simulink model "rlOvertakeTwoCars"  (R2022b)
settings: Solver=ode45  StartTime=0.0  StopTime=inf  FixedStep=0.001  RelTol=5e-3
PreLoadFcn:
  | setUpModel
PostLoadFcn:
  | setUpMain
model workspace (MAT data in the model file):
  firstWarning = 0
  originalScenarioChecksum = 'F73A6DA3C723D3CA73A6F931B7A52A9C'
values from neighbouring files (symbols this model uses):
  accel_vec = (-4:0.5:4)'    [setUpModel.m]
  amax = 3    [setUpMain.m]
  amin = -3    [setUpMain.m]
  dyNorm = [dyNorm 1.1]    [setUpSlipstream.m]
  e1_initial = 0    [setUpMain.m]
  e2_initial = 0    [setUpMain.m]
  L = data.ActorSpecifications.Length    [setUpModel.m]
  psi_o1 = 0.0058 * (pi/180)    (= 0.000101229096616)    [setUpModel.m]
  psi_o2 = 0.3528 *(pi/180)    (= 0.00615752160104)    [setUpModel.m]
  ry = [ry 0]    [setUpSlipstream.m]
  ssSwitch = 1    [setUpSlipstream.m]
  tolpsi = 10 * pi/180    (= 0.174532925199)    [setUpSlipstream.m]
  toly = 1.2*W /2    [setUpSlipstream.m]
  Ts = 0.1    [setUpMPC.m]
  TsRL = Ts    [setUpRLEnv.m]
  umax = 0.3    [setUpMain.m]
  umin = -0.3    [setUpMain.m]
  v_o1 = highSpeed1    (= 35)    [setUpModel.m]
  v_o2 = highSpeed2    (= 36)    [setUpModel.m]
  vel1 = highSpeed1 * ones(length(xlt),length(ylt))    [setUpModel.m]
  vel2 = highSpeed2 * ones(length(xlt),length(ylt))    [setUpModel.m]
  vel_vec = 0:2:20    [setUpModel.m]
  W = data.ActorSpecifications(1,1).Width    [setUpSlipstream.m]
  X_o1 = xRef1(1)    [setUpModel.m]
  X_o2 = xRef2(1)    [setUpModel.m]
  xFollow = [0 x1 xFollow 60]    [setUpSlipstream.m]
  xLead = [0 -x0 xLead]    [setUpSlipstream.m]
  xlt = -250:10:200    [setUpModel.m]
  Y_o1 = yRef1(1)    [setUpModel.m]
  Y_o2 = yRef2(1)    [setUpModel.m]
  yFollow = [c y1 yFollow 1]    [setUpSlipstream.m]
  yLead = [c y0 yLead]    [setUpSlipstream.m]
  ylt = -150:10:100    [setUpModel.m]
undefined symbols (not defined in the file or in its folder): curvature1, curvature2, deg, DiscIntNeverNeededParam, gradbp1, gradbp2, psi, rad, s, v_o, x_colpen, x_o, y_colpen, Z_colpen
libraries: simulink x26, autolibsharedcommon x22, autolibutils x10, autolibshared x10, vehdynlibtirecommon x8, drivingscenarioandsensors x4, autolibpowerinfoutils x4, sharedtransform x4, aerolibconvert2 x2, simulink_extras x2, vehdynlibtire x2, mpcadaslib x1
(part 4 of 8)

== system rlOvertakeTwoCars/Vehicle Body 3DOF Dual Track/sigma ==
  note: 1) Add Subsystem or Model blocks as valid variant choices.
      | 2) You cannot connect blocks at this level. At simulation, connectivity is automatically
      | determined, based on the active variant and port name matching.
  y : Inport
  no sigma : Subsystem  VariantControl=0
  no sigma dual : Subsystem  VariantControl=2
  sigma : Subsystem  VariantControl=1
  sigma dual : Subsystem  VariantControl=3
  alpha_f : Outport  VectorParamsAs1DForOutWhenUnconnected=off
  alpha_r : Outport  Port=2  VectorParamsAs1DForOutWhenUnconnected=off

== system rlOvertakeTwoCars/Vehicle Body 3DOF Dual Track/state ==
  note: 1) Add Subsystem or Model blocks as valid variant choices.
      | 2) You cannot connect blocks at this level. At simulation, connectivity is automatically
      | determined, based on the active variant and port name matching.
  xdot : Inport  Unit=m/s
  xddot_in : Inport  Port=2  PortDimensions=4
  extState : Inport  Port=3
  xdot ext : Subsystem  VariantControl=1
  xdot int : Subsystem  VariantControl=0
  xddot_out : Outport  VectorParamsAs1DForOutWhenUnconnected=off

== system rlOvertakeTwoCars/Vehicle Body 3DOF Dual Track/wind ==
  note: 1) Add Subsystem or Model blocks as valid variant choices.
      | 2) You cannot connect blocks at this level. At simulation, connectivity is automatically
      | determined, based on the active variant and port name matching.
  wind_in : Inport  Unit=m/s
  wind ext : Subsystem  VariantControl=1
  wind int : Subsystem  VariantControl=0
  wind_out : Outport  Unit=m/s  VectorParamsAs1DForOutWhenUnconnected=off

== system rlOvertakeTwoCars/Vehicle Body 3DOF Dual Track Ego/Cy ==
  note: 1) Add Subsystem or Model blocks as valid variant choices.
      | 2) You cannot connect blocks at this level. At simulation, connectivity is automatically
      | determined, based on the active variant and port name matching.
  alpha_f : Inport
  alpha_r : Inport  Port=2
  Cy const : Subsystem  VariantControl=0
  Cy const dual : Subsystem  VariantControl=2
  Cy table : Subsystem  VariantControl=1
  Cy table dual : Subsystem  VariantControl=3
  Cy_f : Outport  VectorParamsAs1DForOutWhenUnconnected=off
  Cy_r : Outport  Port=2  VectorParamsAs1DForOutWhenUnconnected=off

== system rlOvertakeTwoCars/Vehicle Body 3DOF Dual Track Ego/Drag ==
  wind : Inport
  y : Inport  Port=2
  Temp : Inport  Port=3  Unit=K
  Constant : Constant  Value=0
  Demux : Demux  Outputs=3
  Drag Force : autolibsharedcommon/Vehicle Body 3dof/Drag Force  A=Af  beta_w=beta_w  Cd=Cd  Cs=Cs  Cl=Cl  Cpm=Cpm  Lcpm=a+b  Crm=beta_w.*0  Cym=Cym  R=287.058  Pabs=Pabs
  Selector2 : Selector  InputPortWidth=4  IndexOptions=Index vector (dialog)  Indices=[1:3]  OutputSizes=1
  Unary Minus : UnaryMinus
  Unary Minus1 : UnaryMinus
  Vector Concatenate1 : Concatenate  NumInputs=3
  inertial2body : Subsystem
  Fd : Outport  VectorParamsAs1DForOutWhenUnconnected=off
  Md : Outport  Port=2  VectorParamsAs1DForOutWhenUnconnected=off
  wires:
  Temp/1 -> Drag Force/3
  inertial2body/1(Windxyz) -> Drag Force/2
  wind/1 -> inertial2body/2(WindXYZ)
  Demux/3 -> inertial2body/1(psi)
  Demux/1 -> Vector Concatenate1/1
  Demux/2 -> Vector Concatenate1/2
  Constant/1 -> Vector Concatenate1/3
  Vector Concatenate1/1 -> Drag Force/1
  Selector2/1 -> Demux/1
  Drag Force/2 -> Unary Minus1/1
  y/1 -> Selector2/1
  Drag Force/1 -> Unary Minus/1
  Unary Minus/1 -> Fd/1
  Unary Minus1/1 -> Md/1

== system rlOvertakeTwoCars/Vehicle Body 3DOF Dual Track Ego/Signal Routing ==
  note: 1) Add Subsystem or Model blocks as valid variant choices.
      | 2) You cannot connect blocks at this level. At simulation, connectivity is automatically
      | determined, based on the active variant and port name matching.
  y : Inport
  Fbody : Inport  Port=2  Unit=N
  MTotal : Inport  Port=3  Unit=N*m
  FOut : Inport  Port=4
  FTire : Inport  Port=5  Unit=N
  Fg : Inport  Port=6  Unit=N
  FDrag : Inport  Port=7  Unit=N
  MDrag : Inport  Port=8  Unit=N*m
  FExt : Inport  Port=9  Unit=N
  MExt : Inport  Port=10  Unit=N*m
  x : Inport  Port=11
  WhlAngF : Inport  Port=12
  WhlAngR : Inport  Port=13
  Fh : Inport  Port=14  Unit=N
  Mh : Inport  Port=15  Unit=N*m
  Xo : Inport  Port=16
  Signal Routing : Subsystem  VariantControl=0
  Signal Routing Dual : Subsystem  VariantControl=1
  Info : Outport  VectorParamsAs1DForOutWhenUnconnected=off
  xdot : Outport  Port=2  VectorParamsAs1DForOutWhenUnconnected=off
  ydot : Outport  Port=3  VectorParamsAs1DForOutWhenUnconnected=off
  psi : Outport  Port=4  VectorParamsAs1DForOutWhenUnconnected=off
  r : Outport  Port=5  VectorParamsAs1DForOutWhenUnconnected=off
  FzF : Outport  Port=6  VectorParamsAs1DForOutWhenUnconnected=off
  FzR : Outport  Port=7  VectorParamsAs1DForOutWhenUnconnected=off

== system rlOvertakeTwoCars/Vehicle Body 3DOF Dual Track Ego/Slipstream drag multiplier ==
  note: Switch
  note: Lateral offset effect
  note: Drag coefficient ratio
  G : Inport
  Add : Sum  Inputs=-++
  Constant : Constant
  Constant1 : Constant
  "G<0, following" : Lookup_n-D  NumberOfTableDimensions=1  BreakpointsForDimension1=xFollow  Table=yFollow  InternalRulePriority=Speed  RndMeth=Simplest
  "G>0, leading" : Lookup_n-D  NumberOfTableDimensions=1  BreakpointsForDimension1=xLead  Table=yLead  InternalRulePriority=Speed  RndMeth=Simplest
  Lateral multiplier : Lookup_n-D  NumberOfTableDimensions=1  BreakpointsForDimension1=dyNorm  Table=ry  InternalRulePriority=Speed  RndMeth=Simplest
  Multiply : Gain  Gain=-1
  Product : Product
  Switch : Switch  Criteria=u2 > Threshold  SaturateOnIntegerOverflow=off  InputSameDT=off
  Switch1 : Switch  Criteria=u2 > Threshold  SaturateOnIntegerOverflow=off  InputSameDT=off
  r_Cd' : Outport
  tag scope: ry2=global
  wires:
  G/1 -> "G>0, leading"/1, Switch/2, Multiply/1
  "G>0, leading"/1 -> Switch/1
  "G<0, following"/1 -> Switch/3
  Multiply/1 -> "G<0, following"/1
  Constant/1 -> Switch1/3
  Switch1/1 -> r_Cd'/1
  [SsOn] -> Switch1/2
  [dyNorm] -> Lateral multiplier/1
  Switch/1 -> Product/2  "r_Cd"
  Lateral multiplier/1 -> [ry2], Add/1, Product/1  "ry"
  Product/1 -> Add/2
  Constant1/1 -> Add/3
  Add/1 -> Switch1/1

== system rlOvertakeTwoCars/Vehicle Body 3DOF Dual Track Ego/friction ==
  note: 1) Add Subsystem or Model blocks as valid variant choices.
      | 2) You cannot connect blocks at this level. At simulation, connectivity is automatically
      | determined, based on the active variant and port name matching.
  mu_in : Inport  Unit=1
  mu ext : Subsystem  VariantControl=1
  mu ext dual : Subsystem  VariantControl=3
  mu int : Subsystem  VariantControl=0
  mu int dual : Subsystem  VariantControl=2
  mu_out : Outport  Unit=1  VectorParamsAs1DForOutWhenUnconnected=off

== system rlOvertakeTwoCars/Vehicle Body 3DOF Dual Track Ego/front forces ==
  note: 1) Add Subsystem or Model blocks as valid variant choices.
      | 2) You cannot connect blocks at this level. At simulation, connectivity is automatically
      | determined, based on the active variant and port name matching.
  F_in : Inport  Unit=N
  ext : Subsystem  VariantControl=2
  ext dual : Subsystem  VariantControl=5
  ext long : Subsystem  VariantControl=1
  ext long dual : Subsystem  VariantControl=4
  int : Subsystem  VariantControl=0
  int dual : Subsystem  VariantControl=3
  F_out : Outport  Unit=N  VectorParamsAs1DForOutWhenUnconnected=off

== system rlOvertakeTwoCars/Vehicle Body 3DOF Dual Track Ego/front steer ==
  note: 1) Add Subsystem or Model blocks as valid variant choices.
      | 2) You cannot connect blocks at this level. At simulation, connectivity is automatically
      | determined, based on the active variant and port name matching.
  delta_in : Inport  Unit=rad
  delta ext : Subsystem  VariantControl=1
  delta ext dual : Subsystem  VariantControl=3
  delta int : Subsystem  VariantControl=0
  delta int dual : Subsystem  VariantControl=2
  delta_out : Outport  Unit=rad  VectorParamsAs1DForOutWhenUnconnected=off

== system rlOvertakeTwoCars/Vehicle Body 3DOF Dual Track Ego/hitch geometry parameters ==
  note: 1) Add Subsystem or Model blocks as valid variant choices.
      | 2) You cannot connect blocks at this level. At simulation, connectivity is automatically
      | determined, based on the active variant and port name matching.
  hitch active bicycle : Subsystem  VariantControl=1
  hitch active dual track : Subsystem  VariantControl=2
  hitch inactive : Subsystem  VariantControl=3
  dh_out : Outport  Unit=m  VectorParamsAs1DForOutWhenUnconnected=off
  hl_out : Outport  Port=2  Unit=m  VectorParamsAs1DForOutWhenUnconnected=off
  hh_out : Outport  Port=3  Unit=m  VectorParamsAs1DForOutWhenUnconnected=off

== system rlOvertakeTwoCars/Vehicle Body 3DOF Dual Track Ego/sigma ==
  note: 1) Add Subsystem or Model blocks as valid variant choices.
      | 2) You cannot connect blocks at this level. At simulation, connectivity is automatically
      | determined, based on the active variant and port name matching.
  y : Inport
  no sigma : Subsystem  VariantControl=0
  no sigma dual : Subsystem  VariantControl=2
  sigma : Subsystem  VariantControl=1
  sigma dual : Subsystem  VariantControl=3
  alpha_f : Outport  VectorParamsAs1DForOutWhenUnconnected=off
  alpha_r : Outport  Port=2  VectorParamsAs1DForOutWhenUnconnected=off

== system rlOvertakeTwoCars/Vehicle Body 3DOF Dual Track Ego/state ==
  note: 1) Add Subsystem or Model blocks as valid variant choices.
      | 2) You cannot connect blocks at this level. At simulation, connectivity is automatically
      | determined, based on the active variant and port name matching.
  xdot : Inport  Unit=m/s
  xddot_in : Inport  Port=2  PortDimensions=4
  extState : Inport  Port=3
  xdot ext : Subsystem  VariantControl=1
  xdot int : Subsystem  VariantControl=0
  xddot_out : Outport  VectorParamsAs1DForOutWhenUnconnected=off

== system rlOvertakeTwoCars/Vehicle Body 3DOF Dual Track Ego/wind ==
  note: 1) Add Subsystem or Model blocks as valid variant choices.
      | 2) You cannot connect blocks at this level. At simulation, connectivity is automatically
      | determined, based on the active variant and port name matching.
  wind_in : Inport  Unit=m/s
  wind ext : Subsystem  VariantControl=1
  wind int : Subsystem  VariantControl=0
  wind_out : Outport  Unit=m/s  VectorParamsAs1DForOutWhenUnconnected=off

== system rlOvertakeTwoCars/Powertrain & Driveline/Brakes and Wheels/Whl2Veh ==
  FxWhlFrm : Inport  PortDimensions=4
  FyWhlFrm : Inport  Port=2  PortDimensions=4
  WhlAng : Inport  Port=3
  Add : Sum  Inputs=+-
  Add1 : Sum
  Demux2 : Demux  Outputs=[2 2]
  Demux3 : Demux  Outputs=[2 2]
  Product{1..4} (4 alike) : Product
  SinCos : Trigonometry  Operator=sincos
  Vector Concatenate : Concatenate  Mode=Multidimensional array  ConcatenateDimension=2
  Vector Concatenate1 : Concatenate  Mode=Multidimensional array  ConcatenateDimension=2
  FrontF : Outport
  RearF : Outport  Port=2
  wires:
  Vector Concatenate/1 -> FrontF/1
  Demux3/1 -> Vector Concatenate/2
  Demux2/1 -> Vector Concatenate/1
  Demux2/2 -> Vector Concatenate1/1
  Demux3/2 -> Vector Concatenate1/2
  Vector Concatenate1/1 -> RearF/1
  Product4/1 -> Add1/2
  Add/1 -> Demux2/1
  Product2/1 -> Add/2
  SinCos/1 -> Product2/2, Product3/2
  Product1/1 -> Add/1
  SinCos/2 -> Product4/2, Product1/2
  FyWhlFrm/1 -> Product4/1, Product2/1
  Add1/1 -> Demux3/1
  FxWhlFrm/1 -> Product3/1, Product1/1
  Product3/1 -> Add1/1
  WhlAng/1 -> SinCos/1

== system rlOvertakeTwoCars/Powertrain & Driveline/Brakes and Wheels/scale factors with friction ==
  lamda_mu_x : Inport
  lamda_mu_y : Inport  Port=2
  0 : Constant  Value=[zeros(1,numWheels)]  VectorParams1D=off
  Reshape : Reshape  OutputDimensionality=Row vector (2-D)  OutputDimensions=[1,numWheels]
  Reshape1 : Reshape  OutputDimensionality=Row vector (2-D)  OutputDimensions=[1,numWheels]
  Signal Specification3 : SignalSpecification  Unit=1
  Vector Concatenate : Concatenate  NumInputs=5  Mode=Multidimensional array
  ones : Constant  Value=[ones(23,numWheels)]  VectorParams1D=off
  ones2 : Constant  Value=ones(1,numWheels)  VectorParams1D=off
  lambdas : Outport  Unit=1  VectorParamsAs1DForOutWhenUnconnected=off
  wires:
  Signal Specification3/1 -> lambdas/1
  Reshape/1 -> Vector Concatenate/2
  Reshape1/1 -> Vector Concatenate/3
  0/1 -> Vector Concatenate/4  "lamda_mu_V"
  ones/1 -> Vector Concatenate/5
  Vector Concatenate/1 -> Signal Specification3/1
  ones2/1 -> Vector Concatenate/1  "lambda_Fz0"
  lamda_mu_x/1 -> Reshape/1
  lamda_mu_y/1 -> Reshape1/1

== system rlOvertakeTwoCars/Powertrain & Driveline/Vehicle to Tire/Veh2Whl ==
  note: Coordinate Transformation from Axle Fixed Frame to Wheel Fixed Frame
  Vx : Inport
  Vy : Inport  Port=2
  WhlAng : Inport  Port=3
  Add2 : Sum
  Add3 : Sum  Inputs=-+
  Product{5..8} (4 alike) : Product
  SinCos : Trigonometry  Operator=sincos
  VxWhlFrm : Outport
  VyWhlFrm : Outport  Port=2
  wires:
  Add2/1 -> VxWhlFrm/1
  Add3/1 -> VyWhlFrm/1
  Product7/1 -> Add3/1
  Vy/1 -> Product8/1, Product6/1
  SinCos/2 -> Product8/2, Product5/2
  SinCos/1 -> Product7/2, Product6/2
  Product5/1 -> Add2/1
  Product6/1 -> Add2/2
  Product8/1 -> Add3/2
  Vx/1 -> Product5/1, Product7/1
  WhlAng/1 -> SinCos/1

== system rlOvertakeTwoCars/Powertrain & Driveline Ego/Brakes and Wheels/Whl2Veh ==
  FxWhlFrm : Inport  PortDimensions=4
  FyWhlFrm : Inport  Port=2  PortDimensions=4
  WhlAng : Inport  Port=3
  Add : Sum  Inputs=+-
  Add1 : Sum
  Demux2 : Demux  Outputs=[2 2]
  Demux3 : Demux  Outputs=[2 2]
  Product{1..4} (4 alike) : Product
  SinCos : Trigonometry  Operator=sincos
  Vector Concatenate : Concatenate  Mode=Multidimensional array  ConcatenateDimension=2
  Vector Concatenate1 : Concatenate  Mode=Multidimensional array  ConcatenateDimension=2
  FrontF : Outport
  RearF : Outport  Port=2
  wires:
  Vector Concatenate/1 -> FrontF/1
  Demux3/1 -> Vector Concatenate/2
  Demux2/1 -> Vector Concatenate/1
  Demux2/2 -> Vector Concatenate1/1
  Demux3/2 -> Vector Concatenate1/2
  Vector Concatenate1/1 -> RearF/1
  Product4/1 -> Add1/2
  Add/1 -> Demux2/1
  Product2/1 -> Add/2
  SinCos/1 -> Product2/2, Product3/2
  Product1/1 -> Add/1
  SinCos/2 -> Product4/2, Product1/2
  FyWhlFrm/1 -> Product4/1, Product2/1
  Add1/1 -> Demux3/1
  FxWhlFrm/1 -> Product3/1, Product1/1
  Product3/1 -> Add1/1
  WhlAng/1 -> SinCos/1

== system rlOvertakeTwoCars/Powertrain & Driveline Ego/Brakes and Wheels/scale factors with friction ==
  lamda_mu_x : Inport
  lamda_mu_y : Inport  Port=2
  0 : Constant  Value=[zeros(1,numWheels)]  VectorParams1D=off
  Reshape : Reshape  OutputDimensionality=Row vector (2-D)  OutputDimensions=[1,numWheels]
  Reshape1 : Reshape  OutputDimensionality=Row vector (2-D)  OutputDimensions=[1,numWheels]
  Signal Specification3 : SignalSpecification  Unit=1
  Vector Concatenate : Concatenate  NumInputs=5  Mode=Multidimensional array
  ones : Constant  Value=[ones(23,numWheels)]  VectorParams1D=off
  ones2 : Constant  Value=ones(1,numWheels)  VectorParams1D=off
  lambdas : Outport  Unit=1  VectorParamsAs1DForOutWhenUnconnected=off
  wires:
  Signal Specification3/1 -> lambdas/1
  Reshape/1 -> Vector Concatenate/2
  Reshape1/1 -> Vector Concatenate/3
  0/1 -> Vector Concatenate/4  "lamda_mu_V"
  ones/1 -> Vector Concatenate/5
  Vector Concatenate/1 -> Signal Specification3/1
  ones2/1 -> Vector Concatenate/1  "lambda_Fz0"
  lamda_mu_x/1 -> Reshape/1
  lamda_mu_y/1 -> Reshape1/1

== system rlOvertakeTwoCars/Powertrain & Driveline Ego/Vehicle to Tire/Veh2Whl ==
  note: Coordinate Transformation from Axle Fixed Frame to Wheel Fixed Frame
  Vx : Inport
  Vy : Inport  Port=2
  WhlAng : Inport  Port=3
  Add2 : Sum
  Add3 : Sum  Inputs=-+
  Product{5..8} (4 alike) : Product
  SinCos : Trigonometry  Operator=sincos
  VxWhlFrm : Outport
  VyWhlFrm : Outport  Port=2
  wires:
  Add2/1 -> VxWhlFrm/1
  Add3/1 -> VyWhlFrm/1
  Product7/1 -> Add3/1
  Vy/1 -> Product8/1, Product6/1
  SinCos/2 -> Product8/2, Product5/2
  SinCos/1 -> Product7/2, Product6/2
  Product5/1 -> Add2/1
  Product6/1 -> Add2/2
  Product8/1 -> Add3/2
  Vx/1 -> Product5/1, Product7/1
  WhlAng/1 -> SinCos/1

== system rlOvertakeTwoCars/Vehicle Body 3DOF Dual Track/Cy/Cy const ==
  Cyf : Constant  Value=Cy_f
  Cyr : Constant  Value=Cy_r
  Cy_f : Outport  VectorParamsAs1DForOutWhenUnconnected=off
  Cy_r : Outport  Port=2  VectorParamsAs1DForOutWhenUnconnected=off
  wires:
  Cyr/1 -> Cy_r/1
  Cyf/1 -> Cy_f/1

== system rlOvertakeTwoCars/Vehicle Body 3DOF Dual Track/Cy/Cy const dual ==
  Cyf : Constant  Value=Cy_f
  Cyr : Constant  Value=Cy_r
  Vector Concatenate1 : Concatenate
  Vector Concatenate2 : Concatenate  ConcatenateDimension=2
  Cy_f : Outport  VectorParamsAs1DForOutWhenUnconnected=off
  Cy_r : Outport  Port=2  VectorParamsAs1DForOutWhenUnconnected=off
  wires:
  Cyf/1 -> Vector Concatenate2/2, Vector Concatenate2/1
  Cyr/1 -> Vector Concatenate1/2, Vector Concatenate1/1
  Vector Concatenate2/1 -> Cy_f/1
  Vector Concatenate1/1 -> Cy_r/1

== system rlOvertakeTwoCars/Vehicle Body 3DOF Dual Track/Cy/Cy table ==
  alpha_f : Inport
  alpha_r : Inport  Port=2
  Cy_f(alpha_f) : Lookup_n-D  NumberOfTableDimensions=1  BreakpointsForDimension1=alpha_f_brk  Table=Cy_f_data  ExtrapMethod=Clip  InternalRulePriority=Speed  RndMeth=Simplest
  Cy_r(alpha_r) : Lookup_n-D  NumberOfTableDimensions=1  BreakpointsForDimension1=alpha_r_brk  Table=Cy_r_data  ExtrapMethod=Clip  InternalRulePriority=Speed  RndMeth=Simplest
  Cy_f : Outport  VectorParamsAs1DForOutWhenUnconnected=off
  Cy_r : Outport  Port=2  VectorParamsAs1DForOutWhenUnconnected=off
  wires:
  alpha_r/1 -> Cy_r(alpha_r)/1
  alpha_f/1 -> Cy_f(alpha_f)/1
  Cy_r(alpha_r)/1 -> Cy_r/1
  Cy_f(alpha_f)/1 -> Cy_f/1

== system rlOvertakeTwoCars/Vehicle Body 3DOF Dual Track/Cy/Cy table dual ==
  alpha_f : Inport
  alpha_r : Inport  Port=2
  For Each Subsystem : Subsystem  TreatAsAtomicUnit=on
  Cy_f : Outport  VectorParamsAs1DForOutWhenUnconnected=off
  Cy_r : Outport  Port=2  VectorParamsAs1DForOutWhenUnconnected=off
  wires:
  alpha_r/1 -> For Each Subsystem/2(alpha_r)
  alpha_f/1 -> For Each Subsystem/1(alpha_f)
  For Each Subsystem/2(Cy_r) -> Cy_r/1
  For Each Subsystem/1(Cy_f) -> Cy_f/1

== system rlOvertakeTwoCars/Vehicle Body 3DOF Dual Track/Drag/inertial2body ==
  psi : Inport
  WindXYZ : Inport  Port=2
  Add : Sum
  Add1 : Sum  Inputs=-+
  Demux1 : Demux  Outputs=3
  Product{,1..3} (4 alike) : Product
  Trigonometric Function : Trigonometry  Operator=sincos
  Vector Concatenate2 : Concatenate  NumInputs=3
  Windxyz : Outport  VectorParamsAs1DForOutWhenUnconnected=off
  wires:
  psi/1 -> Trigonometric Function/1
  WindXYZ/1 -> Demux1/1
  Product1/1 -> Add/2
  Demux1/3 -> Vector Concatenate2/3
  Product3/1 -> Add/1
  Add/1 -> Vector Concatenate2/1
  Add1/1 -> Vector Concatenate2/2
  Vector Concatenate2/1 -> Windxyz/1
  Product/1 -> Add1/1
  Product2/1 -> Add1/2
  Trigonometric Function/1 -> Product/1, Product1/1
  Trigonometric Function/2 -> Product2/1, Product3/1
  Demux1/1 -> Product/2, Product3/2
  Demux1/2 -> Product1/2, Product2/2

== system rlOvertakeTwoCars/Vehicle Body 3DOF Dual Track/Signal Routing/Signal Routing ==
  y : Inport  PortDimensions=3
  Fbody : Inport  Port=2
  MTotal : Inport  Port=3
  FOut : Inport  Port=4  PortDimensions=6
  FTire : Inport  Port=5
  Fg : Inport  Port=6
  FDrag : Inport  Port=7
  MDrag : Inport  Port=8
  FExt : Inport  Port=9
  MExt : Inport  Port=10
  x : Inport  Port=11
  WhlAngF : Inport  Port=12
  WhlAngR : Inport  Port=13
  Fh : Inport  Port=14
  Mh : Inport  Port=15
  Xo : Inport  Port=16
  Bus Creator17 : BusCreator  Inputs=3
  Bus Selector : BusSelector  OutputSignals=Ang.psi
  Bus Selector1 : BusSelector  OutputSignals=InertFrm
  Bus Selector2 : BusSelector  OutputSignals=BdyFrm
  Demux : Demux  Outputs=3
  Forces 3DOF : Subsystem  VariantControl=2
  Ground : Ground
  Lateral 3DOF : Subsystem  VariantControl=3  mask(Longitudinal 3DOF){aMode=aMode}
  Moments : Subsystem
  Power : Subsystem  VariantControl=3
  Selector : Selector  IndexOptions=Index vector (dialog)  Indices=[1,2,4]  OutputSizes=1
  Signal Specification1 : SignalSpecification  Unit=m/s
  Signal Specification15 : SignalSpecification  Unit=m/s
  Signal Specification2 : SignalSpecification  Unit=rad/s
  Vector Concatenate : Concatenate
  Vector Concatenate1 : Concatenate
  state2bus : Subsystem
  Info : Outport  VectorParamsAs1DForOutWhenUnconnected=off
  xdot : Outport  Port=2  VectorParamsAs1DForOutWhenUnconnected=off
  ydot : Outport  Port=3  VectorParamsAs1DForOutWhenUnconnected=off
  psi : Outport  Port=4  VectorParamsAs1DForOutWhenUnconnected=off
  r : Outport  Port=5  VectorParamsAs1DForOutWhenUnconnected=off
  FzF : Outport  Port=6  VectorParamsAs1DForOutWhenUnconnected=off
  FzR : Outport  Port=7  VectorParamsAs1DForOutWhenUnconnected=off
  wires:
  Fh/1 -> Forces 3DOF/7(Fh)
  FDrag/1 -> Forces 3DOF/2(Fdrag)
  Mh/1 -> Moments/4(Mh)  "Mh"
  Bus Selector/1 -> psi/1  "<psi>"
  Ground/1 -> Power/5(Fsusp)
  Bus Selector2/1 -> Power/2(BodyCg)  "<BdyFrm>"
  Bus Selector1/1 -> Power/1(InertCg)  "<InertFrm>"
  [InfoBus] -> Bus Selector2/1, Bus Selector1/1
  Lateral 3DOF/3(PwrInfo) -> Bus Creator17/3  "PwrInfo"
  Xo/1 -> state2bus/3(Xo)
  Vector Concatenate1/1 -> Lateral 3DOF/7(WhlAngR)
  Vector Concatenate/1 -> Lateral 3DOF/6(WhlAngF)
  WhlAngF/1 -> Vector Concatenate/1, Vector Concatenate/2
  WhlAngR/1 -> Vector Concatenate1/1, Vector Concatenate1/2
  state2bus/2(COM_B) -> Lateral 3DOF/2(BdyFrmCg)  "BdyFrmCg"
  state2bus/1(COM_I) -> Lateral 3DOF/1(InertCg), Bus Selector/1  "InertCg"
  Lateral 3DOF/1(InertFrm) -> Bus Creator17/1  "InertFrm"
  Bus Creator17/1 -> Info/1, [InfoBus]  "Info"
  y/1 -> state2bus/2(y)
  Selector/1 -> Demux/1
  Demux/1 -> Signal Specification15/1
  Demux/2 -> Signal Specification1/1
  Demux/3 -> Signal Specification2/1
  x/1 -> Selector/1, state2bus/1(x)
  Signal Specification15/1 -> xdot/1
  Signal Specification1/1 -> ydot/1
  Signal Specification2/1 -> r/1
  Lateral 3DOF/2(BdyFrm) -> Bus Creator17/2  "BdyFrm"
  Fg/1 -> Forces 3DOF/3(Fg)
  FTire/1 -> Forces 3DOF/6(FTire)
  Forces 3DOF/1(Forces) -> Lateral 3DOF/3(Forces), Power/3(Forces)  "Forces"
  FOut/1 -> Forces 3DOF/4(Fs)
  Forces 3DOF/2(FzF) -> FzF/1
  Forces 3DOF/3(FzR) -> FzR/1
  FExt/1 -> Forces 3DOF/5(Fext)
  Moments/1(Moments) -> Lateral 3DOF/5(Moments), Power/4(Moments)  "Moments"
  MExt/1 -> Moments/3(MExt)  "Ext"
  Power/1(Pwr) -> Lateral 3DOF/4(Power)
  Fbody/1 -> Forces 3DOF/1(FBody)
  MDrag/1 -> Moments/2(Mdrag)  "Drag"
  MTotal/1 -> Moments/1(MBody)

== system rlOvertakeTwoCars/Vehicle Body 3DOF Dual Track/Signal Routing/Signal Routing Dual ==
  y : Inport
  Fbody : Inport  Port=2
  MTotal : Inport  Port=3
  FOut : Inport  Port=4
  FTire : Inport  Port=5
  Fg : Inport  Port=6
  FDrag : Inport  Port=7
  MDrag : Inport  Port=8
  FExt : Inport  Port=9
  MExt : Inport  Port=10
  x : Inport  Port=11
  WhlAngF : Inport  Port=12
  WhlAngR : Inport  Port=13
  Fh : Inport  Port=14
  Mh : Inport  Port=15
  Xo : Inport  Port=16
  Bus Creator17 : BusCreator  Inputs=3
  Bus Selector : BusSelector  OutputSignals=Ang.psi
  Bus Selector1 : BusSelector  OutputSignals=InertFrm
  Bus Selector2 : BusSelector  OutputSignals=BdyFrm
  Demux : Demux  Outputs=3
  Forces 3DOF : Subsystem  VariantControl=2
  Ground : Ground
  Lateral 3DOF : Subsystem  VariantControl=2
  Moments : Subsystem
  Power : Subsystem  VariantControl=4
  Selector : Selector  IndexOptions=Index vector (dialog)  Indices=[1,2,4]  OutputSizes=1
  Signal Specification1 : SignalSpecification  Unit=m/s
  Signal Specification15 : SignalSpecification  Unit=m/s
  Signal Specification2 : SignalSpecification  Unit=rad/s
  state2bus : Subsystem
  Info : Outport  VectorParamsAs1DForOutWhenUnconnected=off
  xdot : Outport  Port=2  VectorParamsAs1DForOutWhenUnconnected=off
  ydot : Outport  Port=3  VectorParamsAs1DForOutWhenUnconnected=off
  psi : Outport  Port=4  VectorParamsAs1DForOutWhenUnconnected=off
  r : Outport  Port=5  VectorParamsAs1DForOutWhenUnconnected=off
  FzF : Outport  Port=6  VectorParamsAs1DForOutWhenUnconnected=off
  FzR : Outport  Port=7  VectorParamsAs1DForOutWhenUnconnected=off
  wires:
  Fh/1 -> Forces 3DOF/7(Fh)
  FTire/1 -> Forces 3DOF/6(FTire)
  Mh/1 -> Moments/4(Mh)  "Mh"
  Bus Selector/1 -> psi/1  "<psi>"
  Demux/3 -> Signal Specification2/1
  Ground/1 -> Power/5(Fsusp)
  Lateral 3DOF/3(PwrInfo) -> Bus Creator17/3  "PwrInfo"
  Bus Selector1/1 -> Power/1(InertCg)  "<InertFrm>"
  [InfoBus] -> Bus Selector2/1, Bus Selector1/1
  Bus Selector2/1 -> Power/2(BodyCg)  "<BdyFrm>"
  Xo/1 -> state2bus/3(Xo)
  WhlAngR/1 -> Lateral 3DOF/7(WhlAngR)
  WhlAngF/1 -> Lateral 3DOF/6(WhlAngF)
  MTotal/1 -> Moments/1(MBody)
  MDrag/1 -> Moments/2(Mdrag)  "Drag"
  Fbody/1 -> Forces 3DOF/1(FBody)
  Power/1(Pwr) -> Lateral 3DOF/4(Power)
  MExt/1 -> Moments/3(MExt)  "Ext"
  Moments/1(Moments) -> Lateral 3DOF/5(Moments), Power/4(Moments)  "Moments"
  FExt/1 -> Forces 3DOF/5(Fext)
  Forces 3DOF/3(FzR) -> FzR/1
  Forces 3DOF/2(FzF) -> FzF/1
  FDrag/1 -> Forces 3DOF/2(Fdrag)
  FOut/1 -> Forces 3DOF/4(Fs)
  Forces 3DOF/1(Forces) -> Lateral 3DOF/3(Forces), Power/3(Forces)  "Forces"
  Fg/1 -> Forces 3DOF/3(Fg)
  Lateral 3DOF/2(BdyFrm) -> Bus Creator17/2  "BdyFrm"
  Signal Specification2/1 -> r/1
  Signal Specification1/1 -> ydot/1
  Signal Specification15/1 -> xdot/1
  x/1 -> Selector/1, state2bus/1(x)
  state2bus/2(COM_B) -> Lateral 3DOF/2(BdyFrmCg)  "BdyFrmCg"
  state2bus/1(COM_I) -> Bus Selector/1, Lateral 3DOF/1(InertCg)  "InertCg"
  Demux/2 -> Signal Specification1/1
  Demux/1 -> Signal Specification15/1
  Selector/1 -> Demux/1
  y/1 -> state2bus/2(y)
  Bus Creator17/1 -> Info/1, [InfoBus]  "Info"
  Lateral 3DOF/1(InertFrm) -> Bus Creator17/1  "InertFrm"

== system rlOvertakeTwoCars/Vehicle Body 3DOF Dual Track/friction/mu ext ==
  mu_in : Inport  Unit=1
  Signal Specification1 : SignalSpecification  Unit=1
  Unit Conversion2 : UnitConversion
  mu_out : Outport  Unit=1  VectorParamsAs1DForOutWhenUnconnected=off
  wires:
  Signal Specification1/1 -> mu_out/1
  mu_in/1 -> Unit Conversion2/1
  Unit Conversion2/1 -> Signal Specification1/1

== system rlOvertakeTwoCars/Vehicle Body 3DOF Dual Track/friction/mu ext dual ==
  mu_in : Inport  PortDimensions=[2,2]
  Signal Specification1 : SignalSpecification  Unit=1
  Unit Conversion2 : UnitConversion
  mu_out : Outport  PortDimensions=[2,2]  VectorParamsAs1DForOutWhenUnconnected=off
  wires:
  Signal Specification1/1 -> mu_out/1
  mu_in/1 -> Unit Conversion2/1
  Unit Conversion2/1 -> Signal Specification1/1

== system rlOvertakeTwoCars/Vehicle Body 3DOF Dual Track/friction/mu int ==
  Constant : Constant  Value=mu
  Vector Concatenate1 : Concatenate
  mu_out : Outport  VectorParamsAs1DForOutWhenUnconnected=off
  wires:
  Constant/1 -> Vector Concatenate1/1, Vector Concatenate1/2
  Vector Concatenate1/1 -> mu_out/1

== system rlOvertakeTwoCars/Vehicle Body 3DOF Dual Track/friction/mu int dual ==
  Constant : Constant  Value=mu
  Vector Concatenate2 : Concatenate  Mode=Multidimensional array  ConcatenateDimension=2
  Vector Concatenate3 : Concatenate  Mode=Multidimensional array  ConcatenateDimension=2
  Vector Concatenate4 : Concatenate  Mode=Multidimensional array
  mu_out : Outport  VectorParamsAs1DForOutWhenUnconnected=off
  wires:
  Vector Concatenate2/1 -> Vector Concatenate4/1
  Vector Concatenate3/1 -> Vector Concatenate4/2
  Vector Concatenate4/1 -> mu_out/1
  Constant/1 -> Vector Concatenate3/2, Vector Concatenate3/1, Vector Concatenate2/2, Vector Concatenate2/1

== system rlOvertakeTwoCars/Vehicle Body 3DOF Dual Track/front forces/ext ==
  F_in : Inport  PortDimensions=2
  Signal Specification1 : SignalSpecification  Unit=N
  Unit Conversion3 : UnitConversion
  F_out : Outport  Unit=N  VectorParamsAs1DForOutWhenUnconnected=off
  wires:
  Signal Specification1/1 -> F_out/1
  F_in/1 -> Unit Conversion3/1
  Unit Conversion3/1 -> Signal Specification1/1

== system rlOvertakeTwoCars/Vehicle Body 3DOF Dual Track/front forces/ext dual ==
  F_in : Inport  PortDimensions=[2,2]
  Signal Specification1 : SignalSpecification  Unit=N
  Unit Conversion3 : UnitConversion
  F_out : Outport  Unit=N  PortDimensions=[2,2]  VectorParamsAs1DForOutWhenUnconnected=off
  wires:
  Signal Specification1/1 -> F_out/1
  F_in/1 -> Unit Conversion3/1
  Unit Conversion3/1 -> Signal Specification1/1

== system rlOvertakeTwoCars/Vehicle Body 3DOF Dual Track/front forces/ext long ==
  F_in : Inport
  Ground1 : Ground
  Signal Specification : SignalSpecification  Unit=N
  Signal Specification1 : SignalSpecification  Unit=N
  Unit Conversion1 : UnitConversion
  Vector Concatenate1 : Concatenate
  F_out : Outport  Unit=N  VectorParamsAs1DForOutWhenUnconnected=off
  wires:
  Signal Specification/1 -> Vector Concatenate1/2
  F_in/1 -> Unit Conversion1/1
  Vector Concatenate1/1 -> F_out/1
  Ground1/1 -> Signal Specification/1
  Unit Conversion1/1 -> Signal Specification1/1
  Signal Specification1/1 -> Vector Concatenate1/1

== system rlOvertakeTwoCars/Vehicle Body 3DOF Dual Track/front forces/ext long dual ==
  F_in : Inport
  Demux : Demux  Outputs=2
  Ground : Ground
  Signal Specification5 : SignalSpecification  Unit=N
  Unit Conversion2 : UnitConversion  OutputType=Inherit: Inherit via back propagation
  Vector Concatenate1 : Concatenate  Mode=Multidimensional array  ConcatenateDimension=2
  Vector Concatenate2 : Concatenate  Mode=Multidimensional array  ConcatenateDimension=2
  Vector Concatenate3 : Concatenate  Mode=Multidimensional array
  F_out : Outport  Unit=N  VectorParamsAs1DForOutWhenUnconnected=off
  wires:
  Ground/1 -> Vector Concatenate2/2, Vector Concatenate1/2
  Vector Concatenate3/1 -> F_out/1
  Vector Concatenate1/1 -> Vector Concatenate3/1
  Vector Concatenate2/1 -> Vector Concatenate3/2
  Demux/1 -> Vector Concatenate1/1
  Demux/2 -> Vector Concatenate2/1
  Unit Conversion2/1 -> Signal Specification5/1
  Signal Specification5/1 -> Demux/1
  F_in/1 -> Unit Conversion2/1

== system rlOvertakeTwoCars/Vehicle Body 3DOF Dual Track/front forces/int ==
  Ground : Ground
  Vector Concatenate1 : Concatenate
  F_out : Outport  VectorParamsAs1DForOutWhenUnconnected=off
  wires:
  Ground/1 -> Vector Concatenate1/2, Vector Concatenate1/1
  Vector Concatenate1/1 -> F_out/1

== system rlOvertakeTwoCars/Vehicle Body 3DOF Dual Track/front forces/int dual ==
  Ground : Ground
  Vector Concatenate2 : Concatenate  Mode=Multidimensional array  ConcatenateDimension=2
  Vector Concatenate3 : Concatenate  Mode=Multidimensional array  ConcatenateDimension=2
  Vector Concatenate4 : Concatenate  Mode=Multidimensional array
  F_out : Outport  VectorParamsAs1DForOutWhenUnconnected=off
  wires:
  Vector Concatenate2/1 -> Vector Concatenate4/1
  Vector Concatenate3/1 -> Vector Concatenate4/2
  Vector Concatenate4/1 -> F_out/1
  Ground/1 -> Vector Concatenate3/2, Vector Concatenate3/1, Vector Concatenate2/2, Vector Concatenate2/1

== system rlOvertakeTwoCars/Vehicle Body 3DOF Dual Track/front steer/delta ext ==
  delta_in : Inport  Unit=rad
  Signal Specification1 : SignalSpecification  Unit=rad
  Unit Conversion1 : UnitConversion
  delta_out : Outport  VectorParamsAs1DForOutWhenUnconnected=off
  wires:
  Signal Specification1/1 -> delta_out/1
  Unit Conversion1/1 -> Signal Specification1/1
  delta_in/1 -> Unit Conversion1/1

== system rlOvertakeTwoCars/Vehicle Body 3DOF Dual Track/front steer/delta ext dual ==
  delta_in : Inport  PortDimensions=2
  Signal Specification1 : SignalSpecification  Unit=rad
  Unit Conversion2 : UnitConversion
  delta_out : Outport  Unit=rad  PortDimensions=2  VectorParamsAs1DForOutWhenUnconnected=off
  wires:
  Signal Specification1/1 -> delta_out/1
  Unit Conversion2/1 -> Signal Specification1/1
  delta_in/1 -> Unit Conversion2/1

== system rlOvertakeTwoCars/Vehicle Body 3DOF Dual Track/front steer/delta int ==
  Ground : Ground
  delta_out : Outport  VectorParamsAs1DForOutWhenUnconnected=off
  wires:
  Ground/1 -> delta_out/1

== system rlOvertakeTwoCars/Vehicle Body 3DOF Dual Track/front steer/delta int dual ==
  Constant : Constant  Value=0
  Vector Concatenate4 : Concatenate
  delta_out : Outport  VectorParamsAs1DForOutWhenUnconnected=off
  wires:
  Constant/1 -> Vector Concatenate4/1, Vector Concatenate4/2
  Vector Concatenate4/1 -> delta_out/1

== system rlOvertakeTwoCars/Vehicle Body 3DOF Dual Track/hitch geometry parameters/hitch active bicycle ==
  Constant : Constant  Value=dh
  Constant1 : Constant  Value=hh
  Ground : Ground
  dh_out : Outport  VectorParamsAs1DForOutWhenUnconnected=off
  hh_out : Outport  Port=2  VectorParamsAs1DForOutWhenUnconnected=off
  hl_out : Outport  Port=3  VectorParamsAs1DForOutWhenUnconnected=off
  wires:
  Ground/1 -> hl_out/1
  Constant1/1 -> hh_out/1
  Constant/1 -> dh_out/1

== system rlOvertakeTwoCars/Vehicle Body 3DOF Dual Track/hitch geometry parameters/hitch active dual track ==
  Constant : Constant  Value=dh
  Constant1 : Constant  Value=hh
  Constant2 : Constant  Value=hl
  dh_out : Outport  VectorParamsAs1DForOutWhenUnconnected=off
  hh_out : Outport  Port=2  VectorParamsAs1DForOutWhenUnconnected=off
  hl_out : Outport  Port=3  VectorParamsAs1DForOutWhenUnconnected=off
  wires:
  Constant2/1 -> hl_out/1
  Constant1/1 -> hh_out/1
  Constant/1 -> dh_out/1

== system rlOvertakeTwoCars/Vehicle Body 3DOF Dual Track/hitch geometry parameters/hitch inactive ==
  Ground : Ground
  dh_out : Outport  Unit=m  PortDimensions=1  VectorParamsAs1DForOutWhenUnconnected=off
  hh_out : Outport  Port=2  Unit=m  PortDimensions=1  VectorParamsAs1DForOutWhenUnconnected=off
  hl_out : Outport  Port=3  Unit=m  PortDimensions=1  VectorParamsAs1DForOutWhenUnconnected=off
  wires:
  Ground/1 -> dh_out/1, hh_out/1, hl_out/1

== system rlOvertakeTwoCars/Vehicle Body 3DOF Dual Track/sigma/no sigma ==
  y : Inport
  Demux : Demux  Outputs=2
  Selector : Selector  InputPortWidth=4  IndexOptions=Index vector (dialog)  Indices=[1,3]  OutputSizes=1
  alpha_f : Outport  VectorParamsAs1DForOutWhenUnconnected=off
  alpha_r : Outport  Port=2  VectorParamsAs1DForOutWhenUnconnected=off
  wires:
  Demux/2 -> alpha_r/1
  Demux/1 -> alpha_f/1
  Selector/1 -> Demux/1
  y/1 -> Selector/1

== system rlOvertakeTwoCars/Vehicle Body 3DOF Dual Track/sigma/no sigma dual ==
  y : Inport  PortDimensions=8
  Demux : Demux  Outputs=[2,2,4]
  Terminator : Terminator
  alpha_f : Outport  VectorParamsAs1DForOutWhenUnconnected=off
  alpha_r : Outport  Port=2  VectorParamsAs1DForOutWhenUnconnected=off
  wires:
  y/1 -> Demux/1
  Demux/1 -> alpha_f/1
  Demux/2 -> alpha_r/1
  Demux/3 -> Terminator/1

== system rlOvertakeTwoCars/Vehicle Body 3DOF Dual Track/sigma/sigma ==
  y : Inport
  Constant1 : Constant  Value=sigma_f
  Constant2 : Constant  Value=sigma_r
  Demux : Demux
  relaxation front : Subsystem
  relaxation rear : Subsystem
  alpha_f : Outport  VectorParamsAs1DForOutWhenUnconnected=off
  alpha_r : Outport  Port=2  VectorParamsAs1DForOutWhenUnconnected=off
  wires:
  Demux/3 -> relaxation rear/1(alpha)
  y/1 -> Demux/1
  Constant1/1 -> relaxation front/3(sigma)
  Constant2/1 -> relaxation rear/3(sigma)
  Demux/2 -> relaxation front/2(V)
  Demux/4 -> relaxation rear/2(V)
  relaxation rear/1(alpha_sig) -> alpha_r/1
  Demux/1 -> relaxation front/1(alpha)
  relaxation front/1(alpha_sig) -> alpha_f/1

== system rlOvertakeTwoCars/Vehicle Body 3DOF Dual Track/sigma/sigma dual ==
  y : Inport  PortDimensions=8
  Constant1 : Constant  Value=sigma_f
  Constant2 : Constant  Value=sigma_r
  Demux : Demux  Outputs=[4,4]
  Demux1 : Demux  Outputs=[2,2]
  Vector Concatenate : Concatenate  NumInputs=4
  relaxation : Subsystem
  alpha_f : Outport  VectorParamsAs1DForOutWhenUnconnected=off
  alpha_r : Outport  Port=2  VectorParamsAs1DForOutWhenUnconnected=off
  wires:
  relaxation/1(alpha_sig) -> Demux1/1
  Demux/1 -> relaxation/1(alpha)
  Demux/2 -> relaxation/2(V)
  y/1 -> Demux/1
  Constant1/1 -> Vector Concatenate/2, Vector Concatenate/1
  Constant2/1 -> Vector Concatenate/3, Vector Concatenate/4
  Vector Concatenate/1 -> relaxation/3(sigma)
  Demux1/1 -> alpha_f/1
  Demux1/2 -> alpha_r/1

== system rlOvertakeTwoCars/Vehicle Body 3DOF Dual Track/state/xdot ext ==
  xdot : Inport
  xddot_in : Inport  Port=2  PortDimensions=4
  extState : Inport  Port=3
  Integrator : Integrator  InitialConditionSource=external  InitialCondition=[x_o;ydot_o;psi;r_o;x_o;xdot_o]
  Selector : Selector  InputPortWidth=4  IndexOptions=Index vector (dialog)  Indices=[2:4]  OutputSizes=1
  Selector1 : Selector  InputPortWidth=4  IndexOptions=Index vector (dialog)  Indices=[2:4]  OutputSizes=1
  Signal Specification : SignalSpecification  Unit=m/s
  Unit Conversion6 : UnitConversion
  Vector Concatenate : Concatenate
  Vector Concatenate1 : Concatenate
  xddot_out : Outport  VectorParamsAs1DForOutWhenUnconnected=off
  wires:
  Selector1/1 -> Vector Concatenate/2
  extState/1 -> Selector1/1
  xddot_in/1 -> Integrator/1
  Vector Concatenate1/1 -> xddot_out/1
  Selector/1 -> Vector Concatenate1/2
  xdot/1 -> Unit Conversion6/1
  Vector Concatenate/1 -> Integrator/2
  Integrator/1 -> Selector/1
  Unit Conversion6/1 -> Signal Specification/1
  Signal Specification/1 -> Vector Concatenate/1, Vector Concatenate1/1

== system rlOvertakeTwoCars/Vehicle Body 3DOF Dual Track/state/xdot int ==
  xddot_in : Inport  PortDimensions=4
  extState : Inport  Port=2
  Integrator : Integrator  InitialConditionSource=external  InitialCondition=[x_o;ydot_o;psi;r_o;x_o;xdot_o]
  xddot_out : Outport  VectorParamsAs1DForOutWhenUnconnected=off
  wires:
  extState/1 -> Integrator/2
  xddot_in/1 -> Integrator/1
  Integrator/1 -> xddot_out/1

== system rlOvertakeTwoCars/Vehicle Body 3DOF Dual Track/wind/wind ext ==
  wind_in : Inport
  Signal Specification1 : SignalSpecification  Unit=m/s
  Unit Conversion5 : UnitConversion
  wind_out : Outport  Unit=m/s  VectorParamsAs1DForOutWhenUnconnected=off
  wires:
  Signal Specification1/1 -> wind_out/1
  wind_in/1 -> Unit Conversion5/1
  Unit Conversion5/1 -> Signal Specification1/1

== system rlOvertakeTwoCars/Vehicle Body 3DOF Dual Track/wind/wind int ==
  Ground : Ground
  Vector Concatenate1 : Concatenate  NumInputs=3
  wind_out : Outport  Unit=m/s  VectorParamsAs1DForOutWhenUnconnected=off
  wires:
  Ground/1 -> Vector Concatenate1/1, Vector Concatenate1/2, Vector Concatenate1/3
  Vector Concatenate1/1 -> wind_out/1

== system rlOvertakeTwoCars/Vehicle Body 3DOF Dual Track Ego/Cy/Cy const ==
  Cyf : Constant  Value=Cy_f
  Cyr : Constant  Value=Cy_r
  Cy_f : Outport  VectorParamsAs1DForOutWhenUnconnected=off
  Cy_r : Outport  Port=2  VectorParamsAs1DForOutWhenUnconnected=off
  wires:
  Cyr/1 -> Cy_r/1
  Cyf/1 -> Cy_f/1

== system rlOvertakeTwoCars/Vehicle Body 3DOF Dual Track Ego/Cy/Cy const dual ==
  Cyf : Constant  Value=Cy_f
  Cyr : Constant  Value=Cy_r
  Vector Concatenate1 : Concatenate
  Vector Concatenate2 : Concatenate  ConcatenateDimension=2
  Cy_f : Outport  VectorParamsAs1DForOutWhenUnconnected=off
  Cy_r : Outport  Port=2  VectorParamsAs1DForOutWhenUnconnected=off
  wires:
  Cyf/1 -> Vector Concatenate2/2, Vector Concatenate2/1
  Cyr/1 -> Vector Concatenate1/2, Vector Concatenate1/1
  Vector Concatenate2/1 -> Cy_f/1
  Vector Concatenate1/1 -> Cy_r/1

== system rlOvertakeTwoCars/Vehicle Body 3DOF Dual Track Ego/Cy/Cy table ==
  alpha_f : Inport
  alpha_r : Inport  Port=2
  Cy_f(alpha_f) : Lookup_n-D  NumberOfTableDimensions=1  BreakpointsForDimension1=alpha_f_brk  Table=Cy_f_data  ExtrapMethod=Clip  InternalRulePriority=Speed  RndMeth=Simplest
  Cy_r(alpha_r) : Lookup_n-D  NumberOfTableDimensions=1  BreakpointsForDimension1=alpha_r_brk  Table=Cy_r_data  ExtrapMethod=Clip  InternalRulePriority=Speed  RndMeth=Simplest
  Cy_f : Outport  VectorParamsAs1DForOutWhenUnconnected=off
  Cy_r : Outport  Port=2  VectorParamsAs1DForOutWhenUnconnected=off
  wires:
  alpha_r/1 -> Cy_r(alpha_r)/1
  alpha_f/1 -> Cy_f(alpha_f)/1
  Cy_r(alpha_r)/1 -> Cy_r/1
  Cy_f(alpha_f)/1 -> Cy_f/1

== system rlOvertakeTwoCars/Vehicle Body 3DOF Dual Track Ego/Cy/Cy table dual ==
  alpha_f : Inport
  alpha_r : Inport  Port=2
  For Each Subsystem : Subsystem  TreatAsAtomicUnit=on
  Cy_f : Outport  VectorParamsAs1DForOutWhenUnconnected=off
  Cy_r : Outport  Port=2  VectorParamsAs1DForOutWhenUnconnected=off
  wires:
  alpha_r/1 -> For Each Subsystem/2(alpha_r)
  alpha_f/1 -> For Each Subsystem/1(alpha_f)
  For Each Subsystem/2(Cy_r) -> Cy_r/1
  For Each Subsystem/1(Cy_f) -> Cy_f/1

== system rlOvertakeTwoCars/Vehicle Body 3DOF Dual Track Ego/Drag/inertial2body ==
  psi : Inport
  WindXYZ : Inport  Port=2
  Add : Sum
  Add1 : Sum  Inputs=-+
  Demux1 : Demux  Outputs=3
  Product{,1..3} (4 alike) : Product
  Trigonometric Function : Trigonometry  Operator=sincos
  Vector Concatenate2 : Concatenate  NumInputs=3
  Windxyz : Outport  VectorParamsAs1DForOutWhenUnconnected=off
  wires:
  psi/1 -> Trigonometric Function/1
  WindXYZ/1 -> Demux1/1
  Product1/1 -> Add/2
  Demux1/3 -> Vector Concatenate2/3
  Product3/1 -> Add/1
  Add/1 -> Vector Concatenate2/1
  Add1/1 -> Vector Concatenate2/2
  Vector Concatenate2/1 -> Windxyz/1
  Product/1 -> Add1/1
  Product2/1 -> Add1/2
  Trigonometric Function/1 -> Product/1, Product1/1
  Trigonometric Function/2 -> Product2/1, Product3/1
  Demux1/1 -> Product/2, Product3/2
  Demux1/2 -> Product1/2, Product2/2

== system rlOvertakeTwoCars/Vehicle Body 3DOF Dual Track Ego/Signal Routing/Signal Routing ==
  y : Inport  PortDimensions=3
  Fbody : Inport  Port=2
  MTotal : Inport  Port=3
  FOut : Inport  Port=4  PortDimensions=6
  FTire : Inport  Port=5
  Fg : Inport  Port=6
  FDrag : Inport  Port=7
  MDrag : Inport  Port=8
  FExt : Inport  Port=9
  MExt : Inport  Port=10
  x : Inport  Port=11
  WhlAngF : Inport  Port=12
  WhlAngR : Inport  Port=13
  Fh : Inport  Port=14
  Mh : Inport  Port=15
  Xo : Inport  Port=16
  Bus Creator17 : BusCreator  Inputs=3
  Bus Selector : BusSelector  OutputSignals=Ang.psi
  Bus Selector1 : BusSelector  OutputSignals=InertFrm
  Bus Selector2 : BusSelector  OutputSignals=BdyFrm
  Demux : Demux  Outputs=3
  Forces 3DOF : Subsystem  VariantControl=2
  Ground : Ground
  Lateral 3DOF : Subsystem  VariantControl=3  mask(Longitudinal 3DOF){aMode=aMode}
  Moments : Subsystem
  Power : Subsystem  VariantControl=3
  Selector : Selector  IndexOptions=Index vector (dialog)  Indices=[1,2,4]  OutputSizes=1
  Signal Specification1 : SignalSpecification  Unit=m/s
  Signal Specification15 : SignalSpecification  Unit=m/s
  Signal Specification2 : SignalSpecification  Unit=rad/s
  Vector Concatenate : Concatenate
  Vector Concatenate1 : Concatenate
  state2bus : Subsystem
  Info : Outport  VectorParamsAs1DForOutWhenUnconnected=off
  xdot : Outport  Port=2  VectorParamsAs1DForOutWhenUnconnected=off
  ydot : Outport  Port=3  VectorParamsAs1DForOutWhenUnconnected=off
  psi : Outport  Port=4  VectorParamsAs1DForOutWhenUnconnected=off
  r : Outport  Port=5  VectorParamsAs1DForOutWhenUnconnected=off
  FzF : Outport  Port=6  VectorParamsAs1DForOutWhenUnconnected=off
  FzR : Outport  Port=7  VectorParamsAs1DForOutWhenUnconnected=off
  wires:
  Fh/1 -> Forces 3DOF/7(Fh)
  FDrag/1 -> Forces 3DOF/2(Fdrag)
  Mh/1 -> Moments/4(Mh)  "Mh"
  Bus Selector/1 -> psi/1  "<psi>"
  Ground/1 -> Power/5(Fsusp)
  Bus Selector2/1 -> Power/2(BodyCg)  "<BdyFrm>"
  Bus Selector1/1 -> Power/1(InertCg)  "<InertFrm>"
  [InfoBus] -> Bus Selector2/1, Bus Selector1/1
  Lateral 3DOF/3(PwrInfo) -> Bus Creator17/3  "PwrInfo"
  Xo/1 -> state2bus/3(Xo)
  Vector Concatenate1/1 -> Lateral 3DOF/7(WhlAngR)
  Vector Concatenate/1 -> Lateral 3DOF/6(WhlAngF)
  WhlAngF/1 -> Vector Concatenate/1, Vector Concatenate/2
  WhlAngR/1 -> Vector Concatenate1/1, Vector Concatenate1/2
  state2bus/2(COM_B) -> Lateral 3DOF/2(BdyFrmCg)  "BdyFrmCg"
  state2bus/1(COM_I) -> Lateral 3DOF/1(InertCg), Bus Selector/1  "InertCg"
  Lateral 3DOF/1(InertFrm) -> Bus Creator17/1  "InertFrm"
  Bus Creator17/1 -> Info/1, [InfoBus]  "Info"
  y/1 -> state2bus/2(y)
  Selector/1 -> Demux/1
  Demux/1 -> Signal Specification15/1
  Demux/2 -> Signal Specification1/1
  Demux/3 -> Signal Specification2/1
  x/1 -> Selector/1, state2bus/1(x)
  Signal Specification15/1 -> xdot/1
  Signal Specification1/1 -> ydot/1
  Signal Specification2/1 -> r/1
  Lateral 3DOF/2(BdyFrm) -> Bus Creator17/2  "BdyFrm"
  Fg/1 -> Forces 3DOF/3(Fg)
  FTire/1 -> Forces 3DOF/6(FTire)
  Forces 3DOF/1(Forces) -> Lateral 3DOF/3(Forces), Power/3(Forces)  "Forces"
  FOut/1 -> Forces 3DOF/4(Fs)
  Forces 3DOF/2(FzF) -> FzF/1
  Forces 3DOF/3(FzR) -> FzR/1
  FExt/1 -> Forces 3DOF/5(Fext)
  Moments/1(Moments) -> Lateral 3DOF/5(Moments), Power/4(Moments)  "Moments"
  MExt/1 -> Moments/3(MExt)  "Ext"
  Power/1(Pwr) -> Lateral 3DOF/4(Power)
  Fbody/1 -> Forces 3DOF/1(FBody)
  MDrag/1 -> Moments/2(Mdrag)  "Drag"
  MTotal/1 -> Moments/1(MBody)
